simulink model "simulink_08_04_procede"  (R2024a)
settings: Solver=VariableStepAuto  StartTime=0.0  StopTime=600  RelTol=1e-3
StartFcn:
  | out = [];
  | disp(Consigne)
  |             disp(T_init);
  |             if Consigne > T_init
  |                 if T_init < 23
  |                     K1 = 0.007628;
  |                     T1 = 0.01103;
  |                     K2 = 0.03405;
  |                     T2 = 0.03035;
  |                     K3 = 0.04391;
  |                     T3 = 0.04924;
  |                 else
  |                     K1 = 0.00881;
  |                     T1 = 0.01194;
  |                     K2 = 0.02418;
  |                     T2 = 0.02359;
  |                     K3 = 0.04385;
  |                     T3 = 0.04942;
  |                 end
  |             else
  |                 if T_init < 30
  |                     K1 = 0.00751;
  |                     T1 = 0.01415;
  |                     K2 = 0.02291;
  |                     T2 = 0.02201;
  |                     K3 = 0.3512;
  |                     T3 = 0.3473;
  |                 else
  |                     K1 = 0.01043;
  |                     T1 = 0.01371;
  |                     K2 = 0.02568;
  |                     T2 = 0.0256;
  |                     K3 = 0.03719;
  |                     T3 = 0.04271;
  |                 end
  |             end
  |             disp('K1');
  |             disp(K1);
StopFcn:
  | try
  |     enreg = get_param('simulink_1avrilhaha/Simulateur Équipe 5', 'Enregistrement');
  |     nom = get_param('simulink_1avrilhaha/Simulateur Équipe 5', 'Fichier');
  | 
  |     if strcmp(enreg, 'on')
  |         dossier = fileparts(get_param('simulink_1avrilhaha', 'FileName'));
  | 
  |         t = out.tout;
  |         y = out.Fichier;
  | 
  |         n = min(length(t), length(y));
  |         t_cut = t(1:n);
  |         y_cut = y(1:n, :);
  | 
  |         T = table(t_cut, y_cut(:,1), 'VariableNames', {'temps', 'sortie'});
  |         writetable(T, fullfile(dossier, [nom '.csv']));
  |     end
  | catch e
  |     disp(['Erreur exportation: ' e.message]);
  | end
undefined symbols (not defined in the file): B2, B3, R1_1, R1_2, R1_3, Rf_1, Rf_2, Rf_3, Rg_1, Rg_2, Rg_3, V1_1, V1_2, V1_3, V2_1, V2_2, V2_3
libraries: simulink_extras x1
settings Model: Creator=sabri  LastModifiedBy=MABRI236
settings DataIOCC: OutputSaveName=y3

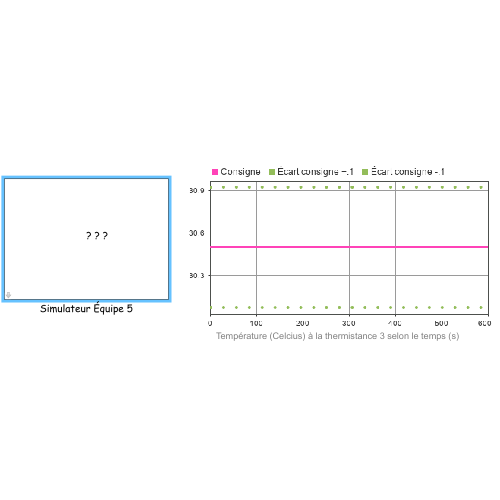
[thumbnail: Simulink's stored preview of the top-level diagram]
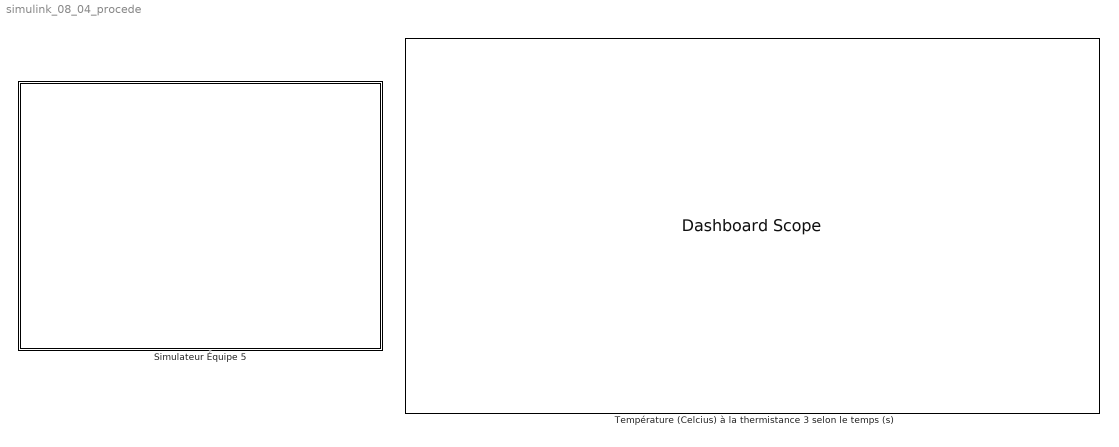
== system simulink_08_04_procede ==
  Simulateur Équipe 5 : Subsystem  mask{Consigne=30.500, T_init=22, Temps=600, Enregistrement=on, Fichier=simulation, V_2=5, V_1=1.8, R_1=3300, R_g=5600, R_f=6300, T_0=298.15, RT_0=10000, B=3900, K1=0, T1=0, K2=0, T2=0, K3=0, T3=0, az=0, bz=0, B1=4100}
      mask prompts: Consigne "Température désirée"; T_init "Température initiale"; Temps "Durée de la simulation (s)"; Enregistrement "Enregistrer les données"; Fichier "Nom du fichier à enregistré:"; V_2 "Tension d'alimentation (V)"; V_1 "Tension d'alimentation de la branche positive de l'ampli-op (V)"; R_1 "Résistance de la branche négative de l'ampli-op (Ω)"; R_g "Résistance en parallèle avec la thermitance (Ω)"; R_f "Résistance du trimpot (Ω)"; T_0 "Température de référence de la thermistance (K)"; RT_0 "Résistance de référence de la thermistance (Ω)"; B "Valeur beta de la thermistance"
      mask DialogControl ParameterGroupVar Prompt: Simulateur
      mask DialogControl Container3 Prompt: Guide d'utilisation
      mask DialogControl Control2 Prompt: Voici le simulateur thermique de l'équipe 5. Vous pouvez modifier les valeurs des différents paramètres du prototype ci-dessus et choisir la température désirée.
      mask DialogControl Control3 Prompt: Lancer la simulation!
      mask DialogControl Container4 Prompt: Paramètres du prototype
      mask DialogControl Container5 Prompt: Thermistance 1
      mask Display: image('4e9b43_37b74c7254004fa5961c1584dfcae1f1~mv2.jpg');
  Température (Celcius) à la thermistance 3 selon le temps (s) : DashboardScope

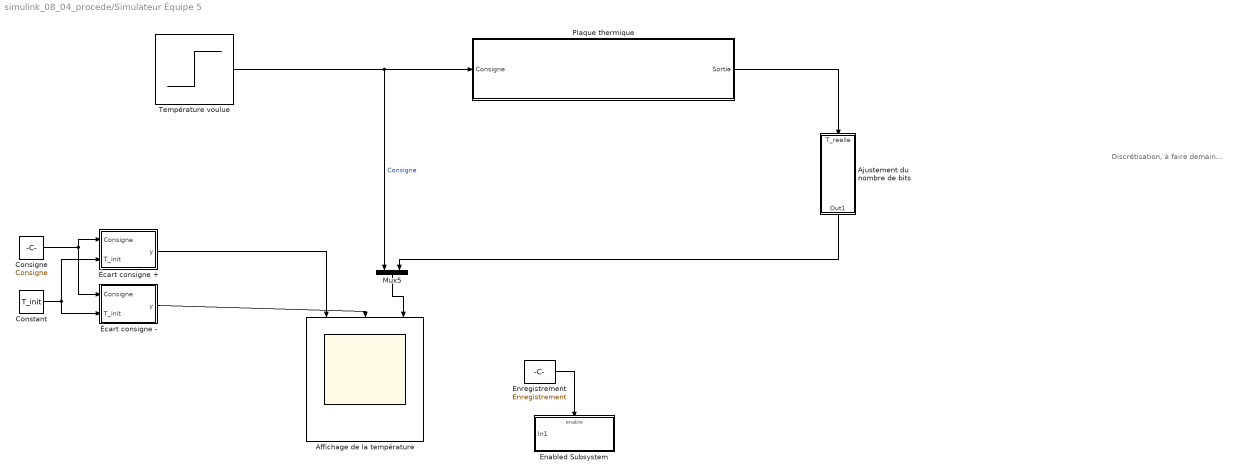
== system simulink_08_04_procede/Simulateur Équipe 5 ==
  note: Discrétisation, à faire demain...
  Affichage de la température : Scope  NumInputPorts=3
  Ajustement du nombre de bits : Subsystem
  Consigne : Constant  Value=Consigne
  Constant : Constant  Value=T_init
  Enabled Subsystem : Subsystem  TreatAsAtomicUnit=on
  Enregistrement : Constant  Value=Enregistrement
  Mux5 : Mux  Inputs=2
  Plaque thermique : Subsystem  TreatAsAtomicUnit=on
  Température voulue : Step  Time=0  Before=T_init  After=Consigne  SampleTime=0
  Écart consigne + : MATLAB Function  TreatAsAtomicUnit=on
  Écart consigne - : MATLAB Function  TreatAsAtomicUnit=on
  wires:
  Écart consigne -/1(y) -> Affichage de la température/2
  Température voulue/1 -> Plaque thermique/1(Consigne), Mux5/1  "Consigne"
  Écart consigne +/1(y) -> Affichage de la température/1
  Enregistrement/1 -> Enabled Subsystem/Enable
  Consigne/1 -> Écart consigne -/1(Consigne), Écart consigne +/1(Consigne)
  Constant/1 -> Écart consigne -/2(T_init), Écart consigne +/2(T_init)
  Mux5/1 -> Affichage de la température/3
  Plaque thermique/1(Sortie) -> Ajustement du nombre de bits/1(T_reelle)
  Ajustement du nombre de bits/1(Out1) -> Mux5/2

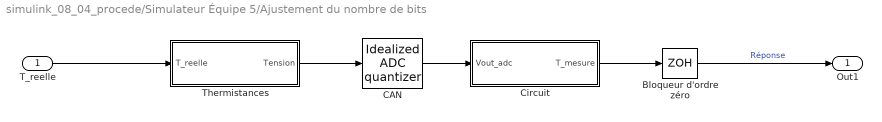
== system simulink_08_04_procede/Simulateur Équipe 5/Ajustement du nombre de bits ==
  T_reelle : Inport
  Bloqueur d'ordre zéro : ZeroOrderHold  SampleTime=0.5
  CAN : simulink_extras/Additional Discrete/Idealized ADC quantizer  NumberOfConverterBits=10  Vmin=0  Vmax=5  OutputDataType=double  OutputNegativeValues=off
  Circuit : Subsystem
  Thermistances : Subsystem
  Out1 : Outport
  wires:
  CAN/1 -> Circuit/1(Vout_adc)
  Circuit/1(T_mesure) -> Bloqueur d'ordre zéro/1
  Thermistances/1(Tension) -> CAN/1
  T_reelle/1 -> Thermistances/1(T_reelle)
  Bloqueur d'ordre zéro/1 -> Out1/1  "Réponse"

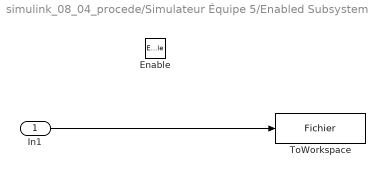
== system simulink_08_04_procede/Simulateur Équipe 5/Enabled Subsystem ==
  In1 : Inport
  Enable : EnablePort
  ToWorkspace : ToWorkspace  VariableName=Fichier  SampleTime=0.5
  wires:
  In1/1 -> ToWorkspace/1

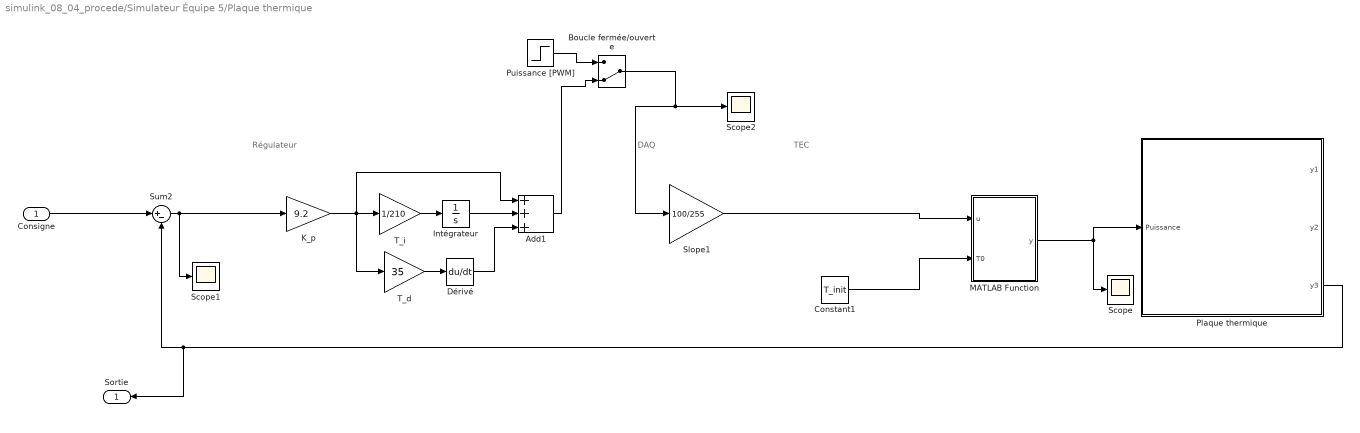
== system simulink_08_04_procede/Simulateur Équipe 5/Plaque thermique ==
  note: Régulateur
  note: DAQ
  note: TEC
  Consigne : Inport
  Add1 : Sum  Inputs=+++
  Boucle fermée/ouverte : ManualSwitch  CurrentSetting=0
  Constant1 : Constant  Value=T_init
  Dérivé : Derivative
  Intégrateur : Integrator
  K_p : Gain  Gain=9.2
  MATLAB Function : MATLAB Function  TreatAsAtomicUnit=on
  Plaque thermique : Subsystem
  Puissance [PWM] : Step  After=-20  SampleTime=0
  Scope : Scope
  Scope1 : Scope
  Scope2 : Scope
  Slope1 : Gain  Gain=100/255
  Sum2 : Sum  Inputs=|+-
  T_d : Gain  Gain=35
  T_i : Gain  Gain=1/210
  Sortie : Outport
  wires:
  Sum2/1 -> Scope1/1, K_p/1
  Intégrateur/1 -> Add1/2
  T_i/1 -> Intégrateur/1
  T_d/1 -> Dérivé/1
  Dérivé/1 -> Add1/3
  K_p/1 -> Add1/1, T_d/1, T_i/1
  Consigne/1 -> Sum2/1
  Constant1/1 -> MATLAB Function/2(T0)
  Slope1/1 -> MATLAB Function/1(u)
  MATLAB Function/1(y) -> Plaque thermique/1(Puissance), Scope/1
  Boucle fermée/ouverte/1 -> Slope1/1, Scope2/1
  Add1/1 -> Boucle fermée/ouverte/2
  Puissance [PWM]/1 -> Boucle fermée/ouverte/1
  Plaque thermique/3(y3) -> Sortie/1, Sum2/2

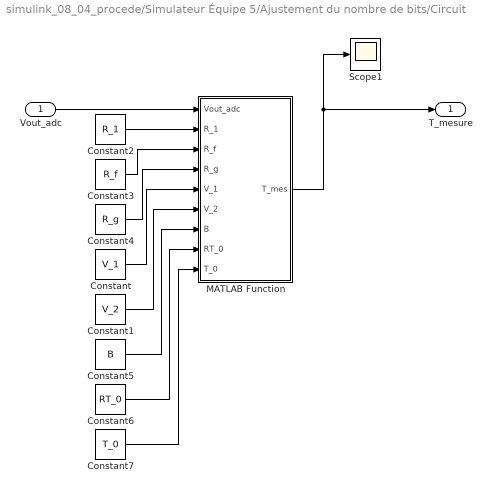
== system simulink_08_04_procede/Simulateur Équipe 5/Ajustement du nombre de bits/Circuit ==
  Vout_adc : Inport
  Constant : Constant  Value=V_1
  Constant1 : Constant  Value=V_2
  Constant2 : Constant  Value=R_1
  Constant3 : Constant  Value=R_f
  Constant4 : Constant  Value=R_g
  Constant5 : Constant  Value=B
  Constant6 : Constant  Value=RT_0
  Constant7 : Constant  Value=T_0
  MATLAB Function : MATLAB Function  TreatAsAtomicUnit=on
  Scope1 : Scope
  T_mesure : Outport
  wires:
  Vout_adc/1 -> MATLAB Function/1(Vout_adc)
  MATLAB Function/1(T_mes) -> Scope1/1, T_mesure/1
  Constant3/1 -> MATLAB Function/3(R_f)
  Constant4/1 -> MATLAB Function/4(R_g)
  Constant7/1 -> MATLAB Function/9(T_0)
  Constant/1 -> MATLAB Function/5(V_1)
  Constant1/1 -> MATLAB Function/6(V_2)
  Constant5/1 -> MATLAB Function/7(B)
  Constant6/1 -> MATLAB Function/8(RT_0)
  Constant2/1 -> MATLAB Function/2(R_1)

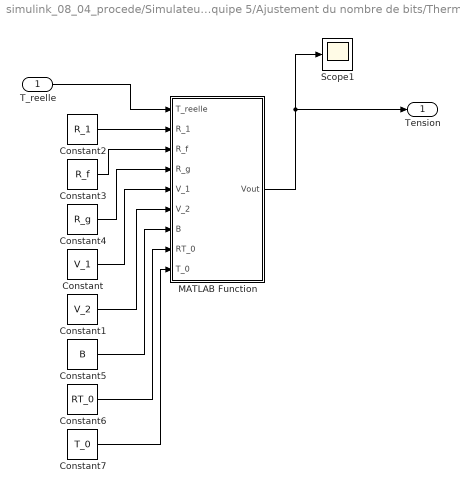
== system simulink_08_04_procede/Simulateur Équipe 5/Ajustement du nombre de bits/Thermistances ==
  T_reelle : Inport
  Constant : Constant  Value=V_1
  Constant1 : Constant  Value=V_2
  Constant2 : Constant  Value=R_1
  Constant3 : Constant  Value=R_f
  Constant4 : Constant  Value=R_g
  Constant5 : Constant  Value=B
  Constant6 : Constant  Value=RT_0
  Constant7 : Constant  Value=T_0
  MATLAB Function : MATLAB Function  TreatAsAtomicUnit=on
  Scope1 : Scope
  Tension : Outport
  wires:
  T_reelle/1 -> MATLAB Function/1(T_reelle)
  MATLAB Function/1(Vout) -> Scope1/1, Tension/1
  Constant7/1 -> MATLAB Function/9(T_0)
  Constant6/1 -> MATLAB Function/8(RT_0)
  Constant5/1 -> MATLAB Function/7(B)
  Constant1/1 -> MATLAB Function/6(V_2)
  Constant/1 -> MATLAB Function/5(V_1)
  Constant4/1 -> MATLAB Function/4(R_g)
  Constant2/1 -> MATLAB Function/2(R_1)
  Constant3/1 -> MATLAB Function/3(R_f)

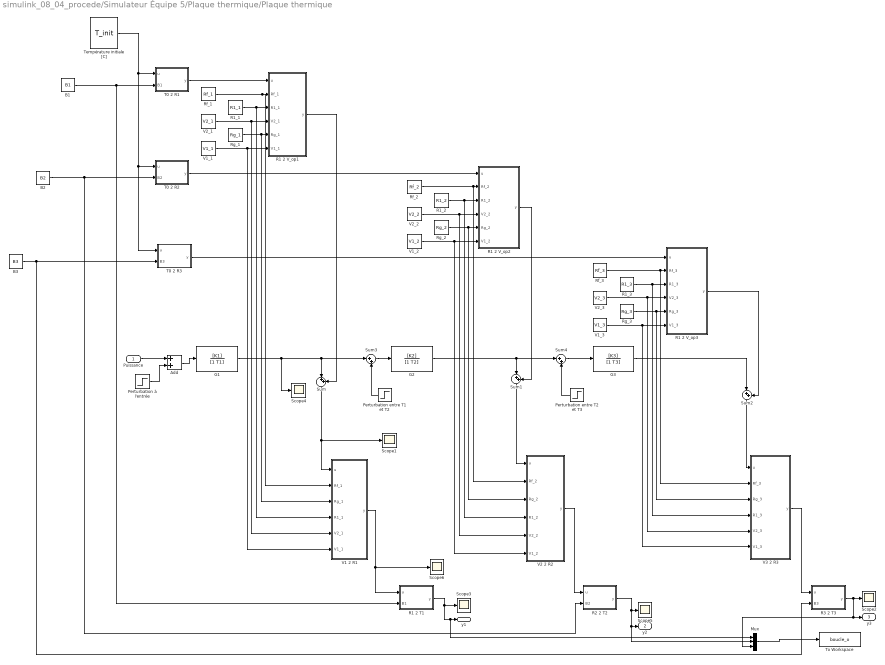
== system simulink_08_04_procede/Simulateur Équipe 5/Plaque thermique/Plaque thermique ==
  Puissance : Inport
  Add : Sum
  B1 : Constant  Value=B1
  B2 : Constant  Value=B2
  B3 : Constant  Value=B3
  G1 : TransferFcn  Numerator=[K1]  Denominator=[1 T1]
  G2 : TransferFcn  Numerator=[K2]  Denominator=[1 T2]
  G3 : TransferFcn  Numerator=[K3]  Denominator=[1 T3]
  Mux : Mux  Inputs=3
  Perturbation entre T1 et T2 : Step  Time=60  After=0  SampleTime=0
  Perturbation entre T2 et T3 : Step  Time=60  After=0  SampleTime=0
  Perturbation à l'entrée : Step  Time=60  After=0  SampleTime=0
  R1 2 T1 : MATLAB Function  TreatAsAtomicUnit=on
  R1 2 V_op1 : MATLAB Function  TreatAsAtomicUnit=on
  R1 2 V_op2 : MATLAB Function  TreatAsAtomicUnit=on
  R1 2 V_op3 : MATLAB Function  TreatAsAtomicUnit=on
  R1_1 : Constant  Value=R1_1
  R1_2 : Constant  Value=R1_2
  R1_3 : Constant  Value=R1_3
  R2 2 T2 : MATLAB Function  TreatAsAtomicUnit=on
  R3 2 T3 : MATLAB Function  TreatAsAtomicUnit=on
  Rf_1 : Constant  Value=Rf_1
  Rf_2 : Constant  Value=Rf_2
  Rf_3 : Constant  Value=Rf_3
  Rg_1 : Constant  Value=Rg_1
  Rg_2 : Constant  Value=Rg_2
  Rg_3 : Constant  Value=Rg_3
  Scope{1..6} (6 alike) : Scope
  Sum{,1..4} (5 alike) : Sum  Inputs=|++
  T0 2 R1 : MATLAB Function  TreatAsAtomicUnit=on
  T0 2 R2 : MATLAB Function  TreatAsAtomicUnit=on
  T0 2 R3 : MATLAB Function  TreatAsAtomicUnit=on
  Température initiale [C] : Constant  Value=T_init
  To Workspace : ToWorkspace  VariableName=boucle_o  SaveFormat=Timeseries  SampleTime=-1
  V1 2 R1 : MATLAB Function  TreatAsAtomicUnit=on
  V1_1 : Constant  Value=V1_1
  V1_2 : Constant  Value=V1_2
  V1_3 : Constant  Value=V1_3
  V2 2 R2 : MATLAB Function  TreatAsAtomicUnit=on
  V2_1 : Constant  Value=V2_1
  V2_2 : Constant  Value=V2_2
  V2_3 : Constant  Value=V2_3
  V3 2 R3 : MATLAB Function  TreatAsAtomicUnit=on
  y1 : Outport
  y2 : Outport  Port=2
  y3 : Outport  Port=3
  wires:
  G2/1 -> Sum1/1, Sum4/1
  R3 2 T3/1(y) -> Mux/3, y3/1, Scope2/1
  V1 2 R1/1(y) -> Scope6/1, R1 2 T1/1(u)
  G3/1 -> Sum2/1
  T0 2 R3/1(y) -> R1 2 V_op3/1(u)
  Sum/1 -> Scope1/1, V1 2 R1/1(u)
  R1 2 V_op1/1(y) -> Sum/2
  Add/1 -> G1/1
  T0 2 R2/1(y) -> R1 2 V_op2/1(u)
  R1 2 V_op3/1(y) -> Sum2/2
  R1 2 V_op2/1(y) -> Sum1/2
  Sum2/1 -> V3 2 R3/1(u)
  T0 2 R1/1(y) -> R1 2 V_op1/1(u)
  R1 2 T1/1(y) -> Mux/1, y1/1, Scope3/1
  Sum1/1 -> V2 2 R2/1(u)
  Température initiale [C]/1 -> T0 2 R3/1(u), T0 2 R2/1(u), T0 2 R1/1(u)
  G1/1 -> Scope4/1, Sum3/1, Sum/1
  Perturbation à l'entrée/1 -> Add/2
  B2/1 -> T0 2 R2/2(B2), R2 2 T2/2(B2)
  B3/1 -> R3 2 T3/2(B3), T0 2 R3/2(B3)
  Puissance/1 -> Add/1
  Sum3/1 -> G2/1
  Sum4/1 -> G3/1
  Perturbation entre T1 et T2/1 -> Sum3/2
  Perturbation entre T2 et T3/1 -> Sum4/2
  V2 2 R2/1(y) -> R2 2 T2/1(u)
  B1/1 -> R1 2 T1/2(B1), T0 2 R1/2(B1)
  R2 2 T2/1(y) -> Mux/2, y2/1, Scope5/1
  Rf_1/1 -> V1 2 R1/2(Rf_1), R1 2 V_op1/2(Rf_1)
  R1_1/1 -> V1 2 R1/4(R1_1), R1 2 V_op1/3(R1_1)
  V2_1/1 -> R1 2 V_op1/4(V2_1), V1 2 R1/5(V2_1)
  Rg_1/1 -> R1 2 V_op1/5(Rg_1), V1 2 R1/3(Rg_1)
  V1_1/1 -> V1 2 R1/6(V1_1), R1 2 V_op1/6(V1_1)
  Rf_2/1 -> V2 2 R2/2(Rf_2), R1 2 V_op2/2(Rf_2)
  R1_2/1 -> V2 2 R2/4(R1_2), R1 2 V_op2/3(R1_2)
  V2_2/1 -> V2 2 R2/5(V2_2), R1 2 V_op2/4(V2_2)
  Rg_2/1 -> V2 2 R2/3(Rg_2), R1 2 V_op2/5(Rg_2)
  V1_2/1 -> V2 2 R2/6(V1_2), R1 2 V_op2/6(V1_2)
  Rf_3/1 -> V3 2 R3/2(Rf_3), R1 2 V_op3/2(Rf_3)
  R1_3/1 -> V3 2 R3/4(R1_3), R1 2 V_op3/3(R1_3)
  V2_3/1 -> V3 2 R3/5(V2_3), R1 2 V_op3/4(V2_3)
  Rg_3/1 -> V3 2 R3/3(Rg_3), R1 2 V_op3/5(Rg_3)
  V1_3/1 -> V3 2 R3/6(V1_3), R1 2 V_op3/6(V1_3)
  V3 2 R3/1(y) -> R3 2 T3/1(u)
  Mux/1 -> To Workspace/1

== matlab function simulink_08_04_procede/Simulateur Équipe 5/Plaque thermique/Plaque thermique/R1 2 T1 ==
  data: u input; y output; B1 input
function y = fcn(u, B1)
disp('B1');
disp(B1);
disp(u);
y = (1/((log(u/10000)/B1)+(1/(298.15))))-273.15;

== matlab function simulink_08_04_procede/Simulateur Équipe 5/Plaque thermique/Plaque thermique/R2 2 T2 ==
  data: u input; y output; B2 input
function y = fcn(u, B2)
y = (1/((log(u/10000)/B2)+(1/(298.15))))-273.15;

== matlab function simulink_08_04_procede/Simulateur Équipe 5/Plaque thermique/Plaque thermique/R3 2 T3 ==
  data: u input; y output; B3 input
function y = fcn(u, B3)

y = (1/((log(u/10000)/B3)+(1/(298.15))))-273.15;

== matlab function simulink_08_04_procede/Simulateur Équipe 5/Plaque thermique/Plaque thermique/T0 2 R1 ==
  data: u input; y output; B1 input
function y = fcn(u, B1)
y = 10000*exp(B1*(1/(u+273.15) - 1/(298.15)));

== matlab function simulink_08_04_procede/Simulateur Équipe 5/Plaque thermique/Plaque thermique/R1 2 V_op1 ==
  data: u input; y output; Rf_1 input; R1_1 input; V2_1 input; Rg_1 input; V1_1 input
function y = fcn_1(u, Rf_1, R1_1, V2_1, Rg_1, V1_1)

y = ((((Rf_1 + R1_1) * Rg_1 * V2_1) / (u + Rg_1)) - Rf_1 * V1_1) / R1_1;

== matlab function simulink_08_04_procede/Simulateur Équipe 5/Plaque thermique/Plaque thermique/R1 2 V_op2 ==
  data: u input; y output; Rf_2 input; R1_2 input; V2_2 input; Rg_2 input; V1_2 input
function y = fcn(u, Rf_2, R1_2, V2_2, Rg_2, V1_2)

y = ((((Rf_2+R1_2)*Rg_2*V2_2)/(u+Rg_2))-Rf_2*V1_2)/R1_2;

== matlab function simulink_08_04_procede/Simulateur Équipe 5/Plaque thermique/Plaque thermique/T0 2 R2 ==
  data: u input; y output; B2 input
function y = fcn(u, B2)
y = 10000*exp(B2*(1/(u+273.15) - 1/(298.15)));

== matlab function simulink_08_04_procede/Simulateur Équipe 5/Plaque thermique/Plaque thermique/R1 2 V_op3 ==
  data: u input; y output; Rf_3 input; R1_3 input; V2_3 input; Rg_3 input; V1_3 input
function y = fcn_3(u, Rf_3, R1_3, V2_3, Rg_3, V1_3)

y = ((((Rf_3 + R1_3) * Rg_3 * V2_3) / (u + Rg_3)) - Rf_3 * V1_3) / R1_3;

== matlab function simulink_08_04_procede/Simulateur Équipe 5/Écart consigne - ==
  data: Consigne input; y output; T_init input
function y = fcn(Consigne, T_init)

y = (-0.05*(Consigne-T_init))+Consigne;

== matlab function simulink_08_04_procede/Simulateur Équipe 5/Plaque thermique/Plaque thermique/T0 2 R3 ==
  data: u input; y output; B3 input
function y = fcn(u, B3)
y = 10000*exp(B3*(1/(u+273.15) - 1/(298.15)));

== matlab function simulink_08_04_procede/Simulateur Équipe 5/Écart consigne + ==
  data: Consigne input; y output; T_init input
function y = fcn(Consigne, T_init)

y = (0.05*(Consigne-T_init))+Consigne;

== matlab function simulink_08_04_procede/Simulateur Équipe 5/Ajustement du nombre de bits/Circuit/MATLAB Function ==
  data: Vout_adc input; T_mes output; R_1 input; R_f input; R_g input; V_1 input; V_2 input; B input; RT_0 input; T_0 input
function T_mes = fcn(Vout_adc, R_1, R_f, R_g, V_1, V_2, B, RT_0, T_0)
    RT = ((R_f + R_1) * R_g * V_2) / (R_1 * (5/1023)*Vout_adc + R_f * V_1) - R_g;
    T_mes = 1.0 / ((log(RT / RT_0) / B) + (1.0 / T_0)) - 273.15;
end

== matlab function simulink_08_04_procede/Simulateur Équipe 5/Plaque thermique/MATLAB Function ==
  data: u input; y output; T0 input
function y = fcn(u, T0)

if u > 0
    y = 0.0022*u^2 -0.0003 * T0^2 + 0.0002 * u * T0 + 0.2083 * u - 0.1342 * T0 + 3.2428;
    disp('puissance chaude');
else
    disp(u);
    y = 0.0048 * u^2 + 0.0001 * T0^2 + 0.0003 * u * T0 + 0.1988 * u - 0.1491 * T0 + 3.3994;
    disp(y);
    disp('puissance froide');


end

== matlab function simulink_08_04_procede/Simulateur Équipe 5/Ajustement du nombre de bits/Thermistances/MATLAB Function ==
  data: T_reelle input; Vout output; R_1 input; R_f input; R_g input; V_1 input; V_2 input; B input; RT_0 input; T_0 input
function Vout = fcn(T_reelle, R_1, R_f, R_g, V_1, V_2, B, RT_0, T_0)
    RT = RT_0 * exp(B * (1/(T_reelle + 273.15) - 1/T_0));
    Vout = ((R_f + R_1) * R_g * V_2) / ((RT + R_g) * R_1) - (R_f * V_1) / R_1;
end

== matlab function simulink_08_04_procede/Simulateur Équipe 5/Plaque thermique/Plaque thermique/V2 2 R2 ==
  data: u input; y output; Rf_2 input; Rg_2 input; R1_2 input; V2_2 input; V1_2 input
function y = fcn_2(u, Rf_2, Rg_2, R1_2, V2_2, V1_2)

% Calcul de la fraction
frac = ((Rf_2 + R1_2) * Rg_2 * V2_2) / (R1_2 * u + Rf_2 * V1_2);

% Vérification : y doit rester positif
if frac - Rg_2 <= 0
    error('fcn_2 : tension u trop élevée, y devient négatif !');
end

% Calcul final
y = frac - Rg_2;

end

== matlab function simulink_08_04_procede/Simulateur Équipe 5/Plaque thermique/Plaque thermique/V1 2 R1 ==
  data: u input; y output; Rf_1 input; Rg_1 input; R1_1 input; V2_1 input; V1_1 input
function y = fcn_1(u, Rf_1, Rg_1, R1_1, V2_1, V1_1)

% Calcul de la fraction
frac = ((Rf_1 + R1_1) * Rg_1 * V2_1) / (R1_1 * u + Rf_1 * V1_1);
disp(Rf_1);
disp(R1_1);
disp(V1_1);
disp(V2_1);
disp(u);

% Vérification : y doit rester positif
if frac - Rg_1 <= 0
    error('fcn_1 : tension u trop élevée, y devient négatif !');
end

% Calcul final
y = frac - Rg_1;

end

== matlab function simulink_08_04_procede/Simulateur Équipe 5/Plaque thermique/Plaque thermique/V3 2 R3 ==
  data: u input; y output; Rf_3 input; Rg_3 input; R1_3 input; V2_3 input; V1_3 input
function y = fcn_3(u, Rf_3, Rg_3, R1_3, V2_3, V1_3)

% Calcul de la fraction
frac = ((Rf_3 + R1_3) * Rg_3 * V2_3) / (R1_3 * u + Rf_3 * V1_3);

% Vérification : y doit rester positif
if frac - Rg_3 <= 0
    error('fcn_3 : tension u trop élevée, y devient négatif !');
end

% Calcul final
y = frac - Rg_3;

end
